simulink model "mdaqdemo_dac2adc_loop"  (R2014a)
settings: Solver=FixedStepDiscrete  SolverMode=SingleTasking  StartTime=0.0  StopTime=inf  FixedStep=0.001  RelTol=1e-3
libraries: microdaq_lib x2
settings Model: SimulationMode=external  CovSFcnEnable=on  ExtModeTrigDuration=10000  Creator=peselnikmg  LastModifiedBy=skibool
settings DataIOCC: SignalLoggingSaveFormat=ModelDataLogs
settings OptimizationCC: OptimizeModelRefInitCode=on  LifeSpan=1
settings DebuggingCC: UnderspecifiedInitializationDetection=Classic  MultiTaskDSMMsg=warning  MultiTaskCondExecSysMsg=none  FrameProcessingCompatibilityMsg=error  StateNameClashWarn=warning
settings HardwareCC: ProdBitPerLong=40  ProdLargestAtomicInteger=Integer  ProdIntDivRoundTo=Zero  ProdEndianess=LittleEndian  ProdHWDeviceType=Texas Instruments->C6000
settings RTWCC: SystemTargetFile=microdaq.tlc  TemplateMakefile=microdaq.tmf  PostCodeGenCommand=microdaq_postcodegen(buildInfo)  Description=MicroDAQ Real-Time Measurement System  GenerateReport=on  IncludeHyperlinkInReport=on
settings CodeAppCC: IgnoreCustomStorageClasses=off
settings STFCustomTargetCC: CodeReplacementLibrary=C89/C90 (ANSI)  ConcurrentExecutionCompliant=off  GeneratePreprocessorConditionals=Use local settings  CombineOutputUpdateFcns=on  ERTCustomFileBanners=on  SupportContinuousTime=off  SupportNonInlinedSFcns=off  MATLABClassNameForMDSCustomization=Simulink.SoftwareTarget.ERTCustomization  GRTInterface=off  SystemTargetFile=microdaq.tlc
settings ERTTargetCC: CodeReplacementLibrary=C89/C90 (ANSI)  GenerateSampleERTMain=off  ExtMode=on  ExtModeStaticAlloc=on  ExtModeStaticAllocSize=1085760  ExtModeMexArgs=getpref('microdaq','TargetIP') 1 4344  InlinedParameterPlacement=Hierarchical  ERTCustomFileTemplate=microdaq_main.tlc

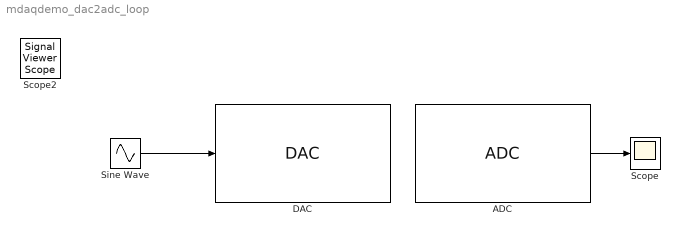
== system mdaqdemo_dac2adc_loop ==
  ADC : microdaq_lib/Analog/ADC  Priority=2  pChannel=1  pChannelCount=ones([1 1 ])  pRange=[-10 10]  pMode=0  pAveraging=Off  SampleTime=0.1
      settings: AttributesFormatString=Priority: %<Priority>
  DAC : microdaq_lib/Analog/DAC  Priority=1  pChannel=1  pChannelCount=ones([1 1 ])  pRange=[0 5]  pInitValue=0  pTermValue=0  pUseInitTerm=2  SampleTime=0.1
      settings: AttributesFormatString=Priority: %<Priority>
  Scope : Scope
      settings: TimeRange=auto  LimitDataPoints=on  MaxDataPoints=5000  SaveToWorkspace=off  SaveName=ScopeData  YMin=1.25  YMax=3.75  SampleTime=-1
  Sine Wave : Sin  Bias=2.5  SampleTime=0.1
      settings: AttributesFormatString=Sample Time: %<SampleTime>
  Scope2 : SignalViewerScope  IOType=viewer  SampleTime=-1  ZoomMode=on
      settings: TimeRange=auto  TickLabels=OneTimeTick  LimitDataPoints=on  SaveToWorkspace=off  SaveName=ScopeData  YMin=-10  YMax=10  SampleInput=off
  wires:
  Sine Wave/1 -> DAC/1
  ADC/1 -> Scope/1
